simulink model "lead_car_appears25a"  (R2025a)
settings: Solver=VariableStepAuto  StartTime=0.0  StopTime=10.0  RelTol=1e-3
settings Model: Creator=jdcjd  LastModifiedBy=jdcjd

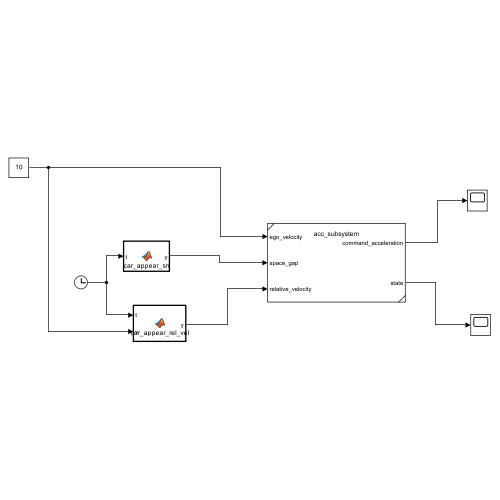
[thumbnail: Simulink's stored preview of the top-level diagram]
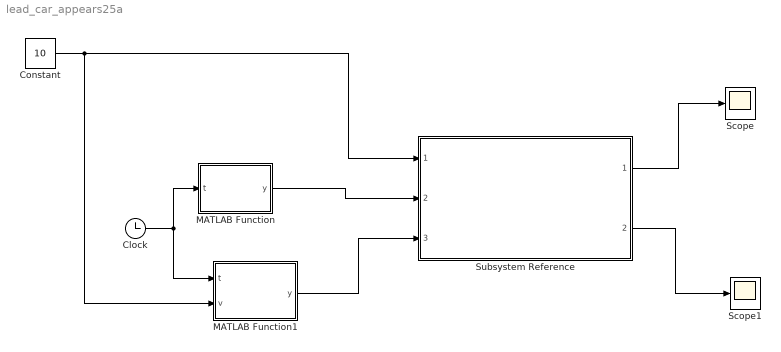
== system lead_car_appears25a ==
  Clock : Clock
  Constant : Constant  Value=10
  MATLAB Function : MATLAB Function  TreatAsAtomicUnit=on
  MATLAB Function1 : MATLAB Function  TreatAsAtomicUnit=on
  Scope : Scope
  Scope1 : Scope
  Subsystem Reference : Subsystem  ReferencedSubsystem=acc_subsystem
  wires:
  Constant/1 -> MATLAB Function1/2(v), Subsystem Reference/1
  Clock/1 -> MATLAB Function/1(t), MATLAB Function1/1(t)
  MATLAB Function/1(y) -> Subsystem Reference/2
  MATLAB Function1/1(y) -> Subsystem Reference/3
  Subsystem Reference/2 -> Scope1/1
  Subsystem Reference/1 -> Scope/1

== matlab function lead_car_appears25a/MATLAB Function ==
  data: t input; y output
function y = car_appear_sn(t)

if t < 3
    y = inf;
else
    y = 15;
end
end

== matlab function lead_car_appears25a/MATLAB Function1 ==
  data: t input; y output; v input
function y = car_appear_rel_vel(t, v)

if t < 3
    y =v;
else 
    y = 8*t -v;
end
end
